simulink model "q7_4"  (R2021a)
settings: Solver=VariableStepAuto  StartTime=0.0  StopTime=10.0  RelTol=1e-3
undefined symbols (not defined in the file or in its folder): a, r, rcos
settings Model: Creator=M__zzZ  LastModifiedBy=M__zzZ

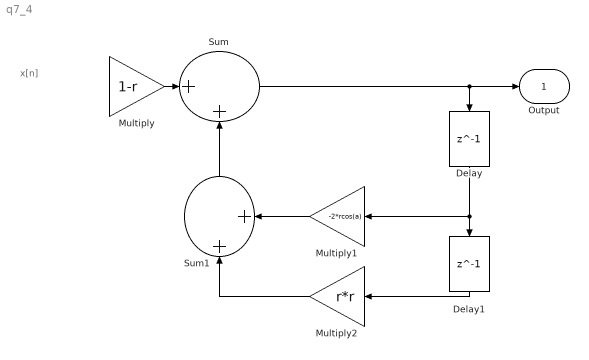
== system q7_4 ==
  note: x[n]
  Delay : Delay  DelayLength=1  InputProcessing=Columns as channels (frame based)
  Delay1 : Delay  DelayLength=1  InputProcessing=Columns as channels (frame based)
  Multiply : Gain  Gain=1-r
  Multiply1 : Gain  Gain=-2*rcos(a)
  Multiply2 : Gain  Gain=r*r
  Sum : Sum  Inputs=|++
  Sum1 : Sum  Inputs=|++
  Output : Outport
  wires:
  Multiply/1 -> Sum/1
  Sum1/1 -> Sum/2
  Multiply1/1 -> Sum1/2
  Multiply2/1 -> Sum1/1
  Delay/1 -> Multiply1/1, Delay1/1
  Delay1/1 -> Multiply2/1
  Sum/1 -> Delay/1, Output/1
